simulink model "testfor122_fun"  (R2016a)
settings: Solver=VariableStepAuto  StartTime=0.0  StopTime=20  RelTol=1e-3
settings Model: Creator=Ping  LastModifiedBy=Ping

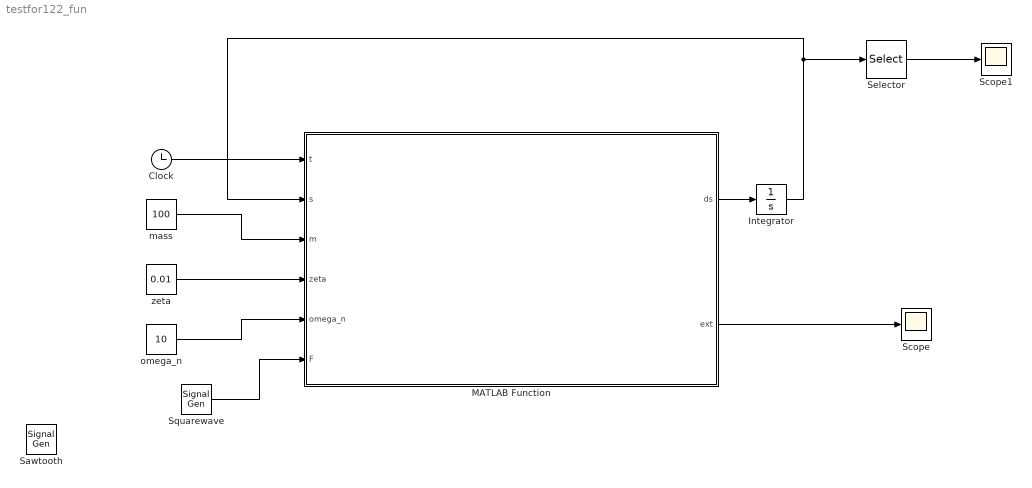
== system testfor122_fun ==
  Clock : Clock
  Integrator : Integrator  InitialCondition=[0.1 0]
  MATLAB Function : MATLAB Function  TreatAsAtomicUnit=on
  "Sawtooth " : SignalGenerator  WaveForm=sawtooth  Amplitude=1000  Frequency=5  Units=rad/sec
  Scope : Scope
  Scope1 : Scope
  Selector : Selector  InputPortWidth=2  IndexOptions=Index vector (dialog)  Indices=[1]  OutputSizes=1
  "Squarewave " : SignalGenerator  WaveForm=square  Units=rad/sec
  mass : Constant  Value=100
  omega_n : Constant  Value=10
  zeta : Constant  Value=0.01
  wires:
  Clock/1 -> MATLAB Function/1(t)
  zeta/1 -> MATLAB Function/4(zeta)
  mass/1 -> MATLAB Function/3(m)
  omega_n/1 -> MATLAB Function/5(omega_n)
  MATLAB Function/1(ds) -> Integrator/1
  Integrator/1 -> MATLAB Function/2(s), Selector/1
  MATLAB Function/2(ext) -> Scope/1
  Selector/1 -> Scope1/1
  "Squarewave "/1 -> MATLAB Function/6(F)

== matlab function testfor122_fun/MATLAB Function ==
  data: t input; ds output; s input; m input; zeta input; omega_n input; F input; ext output
function [ds, ext] = testfor122_fun(t,s,m,zeta,omega_n,F)
%#codegen

x=s(1);
v=s(2);

c=2*m*omega_n*zeta;
k=(omega_n^2)*m;

x_dot=v;
v_dot=(1/m)*(F-c*v-k*x);

ds=[x_dot;v_dot];
ext=F;
